simulink model "gap_generation_single_veh"  (R2019a)
settings: Solver=VariableStepAuto  StartTime=0.0  StopTime=35  FixedStep=0.1  MaxStep=0.05  RelTol=1e-3
libraries: simulink x21, powerlib_meascontrol x5, autolibshared x5
(part 1 of 3)
settings Model: Creator=fvall  LastModifiedBy=fvall

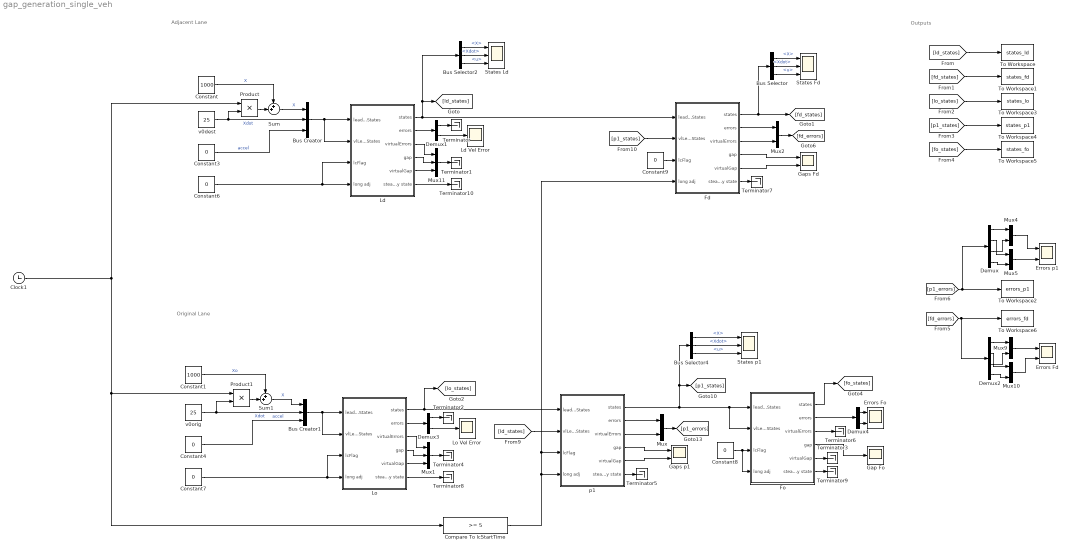
== system gap_generation_single_veh ==
  note: Original Lane
  note: Adjacent Lane
  note: Outputs
  Bus Creator : BusCreator  Inputs=3
  Bus Creator1 : BusCreator  Inputs=3
  Bus Selector : BusSelector  OutputSignals=X,Xdot,u
  Bus Selector2 : BusSelector  OutputSignals=X,Xdot,u
  Bus Selector4 : BusSelector  OutputSignals=X,Xdot,u
  Clock1 : Clock
  Compare To lcStartTime : simulink/Logic and Bit Operations/Compare To Constant  relop=>=  const=5  OutDataTypeStr=boolean
  Constant : Constant  Value=1000
  Constant1 : Constant  Value=1000
  Constant{3..4,6..9} (6 alike) : Constant  Value=0
  Demux : Demux
  Demux1 : Demux  Outputs=2
  Demux2 : Demux
  Demux3 : Demux  Outputs=2
  Demux4 : Demux  Outputs=2
  Errors Fd : Scope  NumInputPorts=2
  Errors Fo : Scope  NumInputPorts=2
  Errors p1 : Scope  NumInputPorts=2
  Fd : Subsystem  mask{m=2000, lf=2.5, lr=2.5, maxAcceleration=4, minAcceleration=-8, maxJerk=40, minJerk=-50, x0=20.2504, vx0=25, y0=3.6, h=0.63, d0=0.5004, minHeadwayError=-100, maxHeadwayError=3, velFilterGain=10, Kd=1.5652, Kp=2.2775, Ki=0.75, velKi=0.5, velKp=1.5, hFilterGain=0.5, vMin=16.25, l1=-10, maxComfAccel=2, minComfAccel=-2, maxComfJerk=10, minComfJerk=-10, hLc=1.9025, d0Lc=0.5004}
      mask prompts: m "autoblks_shared:autoblkVehBody3DofLat:blkPrm_m"; lf "autoblks_shared:autoblkVehBody3DofLat:blkPrm_a"; lr "autoblks_shared:autoblkVehBody3DofLat:blkPrm_b"; maxAcceleration "Max Acceleration"; minAcceleration "Min Acceleration"; maxJerk "Max Jerk"; minJerk "Min Jerk"; x0 "autoblks_shared:autoblkVehBody3DofLat:blkPrm_X_o"; vx0 "autoblks_shared:autoblkVehBody3DofLat:blkPrm_xdot_o"; y0 "autoblks_shared:autoblkVehBody3DofLat:blkPrm_Y_o"; h "Time Headway"; d0 "Standstill Gap"; minHeadwayError "Min Headway Error"; maxHeadwayError "Max Headway Error"; velFilterGain "Velocity Filter Gain"; hFilterGain "Headway filter Gain"; vMin "Min velocity"; l1 "ACC-v Headway Error Threshold"; maxComfAccel "Max Comf Accel"; minComfAccel "Min Comf Accel"; maxComfJerk "Max Comf Jerk"; minComfJerk "Min Comf Jerk"; hLc "Time Headway LC"; d0Lc "Standstill Gap LC"
      mask TypeOptions m: Vehicle Body 3DOF Single Track/m
      mask TypeOptions lf: Vehicle Body 3DOF Single Track/a
      mask TypeOptions lr: Vehicle Body 3DOF Single Track/b
      mask TypeOptions x0: Vehicle Body 3DOF Single Track/X_o
      mask TypeOptions vx0: Vehicle Body 3DOF Single Track/xdot_o
      mask TypeOptions y0: Vehicle Body 3DOF Single Track/Y_o
      mask TypeOptions h:
      | Regular Vehicle
      | Following/Headway error/h/Value
      mask TypeOptions d0:
      | Regular Vehicle
      | Following/Headway error/d0/Value
      mask TypeOptions hFilterGain:
      | Regular Vehicle
      | Following/Headway error/hFilterGain/Gain
      mask TypeOptions vMin:
      | Longitudinal Adjustments
      | for Lane Change/vMin/Value
      mask TypeOptions hLc:
      | Regular Vehicle
      | Following/Headway error/hLc/Value
      mask TypeOptions d0Lc:
      | Regular Vehicle
      | Following/Headway error/d0Lc/Value
      mask DialogControl DescGroupVar Prompt: 3DOF Vehicle with ACC
      mask DialogControl DescTextVar Prompt: Vehicle with ACC. The vehicle model is Simulink's 3DOF single track vehicle body. The controller is a PID with constant headway including headway error saturation and filtered leader velocity.
      mask DialogControl VehParams Prompt: Vehicle Parameters
      mask DialogControl m Prompt: Vehicle mass, m [kg]:
      mask DialogControl lf Prompt: Longitudinal distance from center of mass to front axle, a [m]:
      mask DialogControl lr Prompt: Longitudinal distance from center of mass to rear axle, b [m]:
      mask DialogControl InitStates Prompt: Initial State
      mask DialogControl x0 Prompt: Initial inertial frame longitudinal position, X_o [m]:
      mask DialogControl vx0 Prompt: Initial longitudinal velocity, xdot_o [m/s]:
      mask DialogControl y0 Prompt: Initial inertial frame lateral displacement, Y_o [m]:
      mask DialogControl Container3 Prompt: Veh Following Parameters
      mask DialogControl VirtualFollParams Prompt: Virtual Veh Following Parameters
      mask DialogControl LCParams Prompt: Lane Change Params
  Fo : Subsystem  mask{m=2000, lf=2.5, lr=2.5, maxAcceleration=4, minAcceleration=-8, maxJerk=40, minJerk=-50, x0=0, vx0=25, y0=0, h=0.63, d0=0.5004, minHeadwayError=-100, maxHeadwayError=3, velFilterGain=10, Kd=1.5652, Kp=2.2775, Ki=0.75, velKi=0.5, velKp=1.5, hFilterGain=0.5, vMin=16.25, l1=-10, maxComfAccel=2, minComfAccel=-2, maxComfJerk=10, minComfJerk=-10, hLc=1.9025, d0Lc=0.5004}
      mask prompts: m "autoblks_shared:autoblkVehBody3DofLat:blkPrm_m"; lf "autoblks_shared:autoblkVehBody3DofLat:blkPrm_a"; lr "autoblks_shared:autoblkVehBody3DofLat:blkPrm_b"; maxAcceleration "Max Acceleration"; minAcceleration "Min Acceleration"; maxJerk "Max Jerk"; minJerk "Min Jerk"; x0 "autoblks_shared:autoblkVehBody3DofLat:blkPrm_X_o"; vx0 "autoblks_shared:autoblkVehBody3DofLat:blkPrm_xdot_o"; y0 "autoblks_shared:autoblkVehBody3DofLat:blkPrm_Y_o"; h "Time Headway"; d0 "Standstill Gap"; minHeadwayError "Min Headway Error"; maxHeadwayError "Max Headway Error"; velFilterGain "Velocity Filter Gain"; hFilterGain "Headway filter Gain"; vMin "Min velocity"; l1 "ACC-v Headway Error Threshold"; maxComfAccel "Max Comf Accel"; minComfAccel "Min Comf Accel"; maxComfJerk "Max Comf Jerk"; minComfJerk "Min Comf Jerk"; hLc "Time Headway LC"; d0Lc "Standstill Gap LC"
      mask TypeOptions m: Vehicle Body 3DOF Single Track/m
      mask TypeOptions lf: Vehicle Body 3DOF Single Track/a
      mask TypeOptions lr: Vehicle Body 3DOF Single Track/b
      mask TypeOptions x0: Vehicle Body 3DOF Single Track/X_o
      mask TypeOptions vx0: Vehicle Body 3DOF Single Track/xdot_o
      mask TypeOptions y0: Vehicle Body 3DOF Single Track/Y_o
      mask TypeOptions h:
      | Regular Vehicle
      | Following/Headway error/h/Value
      mask TypeOptions d0:
      | Regular Vehicle
      | Following/Headway error/d0/Value
      mask TypeOptions hFilterGain:
      | Regular Vehicle
      | Following/Headway error/hFilterGain/Gain
      mask TypeOptions vMin:
      | Longitudinal Adjustments
      | for Lane Change/vMin/Value
      mask TypeOptions hLc:
      | Regular Vehicle
      | Following/Headway error/hLc/Value
      mask TypeOptions d0Lc:
      | Regular Vehicle
      | Following/Headway error/d0Lc/Value
      mask DialogControl DescGroupVar Prompt: 3DOF Vehicle with ACC
      mask DialogControl DescTextVar Prompt: Vehicle with ACC. The vehicle model is Simulink's 3DOF single track vehicle body. The controller is a PID with constant headway including headway error saturation and filtered leader velocity.
      mask DialogControl VehParams Prompt: Vehicle Parameters
      mask DialogControl m Prompt: Vehicle mass, m [kg]:
      mask DialogControl lf Prompt: Longitudinal distance from center of mass to front axle, a [m]:
      mask DialogControl lr Prompt: Longitudinal distance from center of mass to rear axle, b [m]:
      mask DialogControl InitStates Prompt: Initial State
      mask DialogControl x0 Prompt: Initial inertial frame longitudinal position, X_o [m]:
      mask DialogControl vx0 Prompt: Initial longitudinal velocity, xdot_o [m/s]:
      mask DialogControl y0 Prompt: Initial inertial frame lateral displacement, Y_o [m]:
      mask DialogControl Container3 Prompt: Veh Following Parameters
      mask DialogControl VirtualFollParams Prompt: Virtual Veh Following Parameters
      mask DialogControl LCParams Prompt: Lane Change Params
  Gap Fo : Scope
  Gaps Fd : Scope  NumInputPorts=2
  Gaps p1 : Scope  NumInputPorts=2
  Ld : Subsystem  mask{m=2000, lf=2.5, lr=2.5, maxAcceleration=4, minAcceleration=-8, maxJerk=40, minJerk=-50, x0=41.5008, vx0=25, y0=3.6, h=0.63, d0=0.5004, minHeadwayError=-100, maxHeadwayError=3, velFilterGain=10, Kd=1.5652, Kp=2.2775, Ki=0.75, velKi=0.5, velKp=1.5, hFilterGain=0.5, vMin=16.25, l1=-10, maxComfAccel=2, minComfAccel=-2, maxComfJerk=10, minComfJerk=-10, hLc=1.9025, d0Lc=0.5004}
      mask prompts: m "autoblks_shared:autoblkVehBody3DofLat:blkPrm_m"; lf "autoblks_shared:autoblkVehBody3DofLat:blkPrm_a"; lr "autoblks_shared:autoblkVehBody3DofLat:blkPrm_b"; maxAcceleration "Max Acceleration"; minAcceleration "Min Acceleration"; maxJerk "Max Jerk"; minJerk "Min Jerk"; x0 "autoblks_shared:autoblkVehBody3DofLat:blkPrm_X_o"; vx0 "autoblks_shared:autoblkVehBody3DofLat:blkPrm_xdot_o"; y0 "autoblks_shared:autoblkVehBody3DofLat:blkPrm_Y_o"; h "Time Headway"; d0 "Standstill Gap"; minHeadwayError "Min Headway Error"; maxHeadwayError "Max Headway Error"; velFilterGain "Velocity Filter Gain"; hFilterGain "Headway filter Gain"; vMin "Min velocity"; l1 "ACC-v Headway Error Threshold"; maxComfAccel "Max Comf Accel"; minComfAccel "Min Comf Accel"; maxComfJerk "Max Comf Jerk"; minComfJerk "Min Comf Jerk"; hLc "Time Headway LC"; d0Lc "Standstill Gap LC"
      mask TypeOptions m: Vehicle Body 3DOF Single Track/m
      mask TypeOptions lf: Vehicle Body 3DOF Single Track/a
      mask TypeOptions lr: Vehicle Body 3DOF Single Track/b
      mask TypeOptions x0: Vehicle Body 3DOF Single Track/X_o
      mask TypeOptions vx0: Vehicle Body 3DOF Single Track/xdot_o
      mask TypeOptions y0: Vehicle Body 3DOF Single Track/Y_o
      mask TypeOptions h:
      | Regular Vehicle
      | Following/Headway error/h/Value
      mask TypeOptions d0:
      | Regular Vehicle
      | Following/Headway error/d0/Value
      mask TypeOptions hFilterGain:
      | Regular Vehicle
      | Following/Headway error/hFilterGain/Gain
      mask TypeOptions vMin:
      | Longitudinal Adjustments
      | for Lane Change/vMin/Value
      mask TypeOptions hLc:
      | Regular Vehicle
      | Following/Headway error/hLc/Value
      mask TypeOptions d0Lc:
      | Regular Vehicle
      | Following/Headway error/d0Lc/Value
      mask DialogControl DescGroupVar Prompt: 3DOF Vehicle with ACC
      mask DialogControl DescTextVar Prompt: Vehicle with ACC. The vehicle model is Simulink's 3DOF single track vehicle body. The controller is a PID with constant headway including headway error saturation and filtered leader velocity.
      mask DialogControl VehParams Prompt: Vehicle Parameters
      mask DialogControl m Prompt: Vehicle mass, m [kg]:
      mask DialogControl lf Prompt: Longitudinal distance from center of mass to front axle, a [m]:
      mask DialogControl lr Prompt: Longitudinal distance from center of mass to rear axle, b [m]:
      mask DialogControl InitStates Prompt: Initial State
      mask DialogControl x0 Prompt: Initial inertial frame longitudinal position, X_o [m]:
      mask DialogControl vx0 Prompt: Initial longitudinal velocity, xdot_o [m/s]:
      mask DialogControl y0 Prompt: Initial inertial frame lateral displacement, Y_o [m]:
      mask DialogControl Container3 Prompt: Veh Following Parameters
      mask DialogControl VirtualFollParams Prompt: Virtual Veh Following Parameters
      mask DialogControl LCParams Prompt: Lane Change Params
  Ld Vel Error : Scope
  Lo : Subsystem  mask{m=2000, lf=2.5, lr=2.5, maxAcceleration=4, minAcceleration=-8, maxJerk=40, minJerk=-50, x0=42.5008, vx0=25, y0=0, h=0.63, d0=0.5004, minHeadwayError=-100, maxHeadwayError=3, velFilterGain=10, Kd=1.5652, Kp=2.2775, Ki=0.75, velKi=0.5, velKp=1.5, hFilterGain=0.5, vMin=16.25, l1=-10, maxComfAccel=2, minComfAccel=-2, maxComfJerk=10, minComfJerk=-10, hLc=1.9025, d0Lc=0.5004}
      mask prompts: m "autoblks_shared:autoblkVehBody3DofLat:blkPrm_m"; lf "autoblks_shared:autoblkVehBody3DofLat:blkPrm_a"; lr "autoblks_shared:autoblkVehBody3DofLat:blkPrm_b"; maxAcceleration "Max Acceleration"; minAcceleration "Min Acceleration"; maxJerk "Max Jerk"; minJerk "Min Jerk"; x0 "autoblks_shared:autoblkVehBody3DofLat:blkPrm_X_o"; vx0 "autoblks_shared:autoblkVehBody3DofLat:blkPrm_xdot_o"; y0 "autoblks_shared:autoblkVehBody3DofLat:blkPrm_Y_o"; h "Time Headway"; d0 "Standstill Gap"; minHeadwayError "Min Headway Error"; maxHeadwayError "Max Headway Error"; velFilterGain "Velocity Filter Gain"; hFilterGain "Headway filter Gain"; vMin "Min velocity"; l1 "ACC-v Headway Error Threshold"; maxComfAccel "Max Comf Accel"; minComfAccel "Min Comf Accel"; maxComfJerk "Max Comf Jerk"; minComfJerk "Min Comf Jerk"; hLc "Time Headway LC"; d0Lc "Standstill Gap LC"
      mask TypeOptions m: Vehicle Body 3DOF Single Track/m
      mask TypeOptions lf: Vehicle Body 3DOF Single Track/a
      mask TypeOptions lr: Vehicle Body 3DOF Single Track/b
      mask TypeOptions x0: Vehicle Body 3DOF Single Track/X_o
      mask TypeOptions vx0: Vehicle Body 3DOF Single Track/xdot_o
      mask TypeOptions y0: Vehicle Body 3DOF Single Track/Y_o
      mask TypeOptions h:
      | Regular Vehicle
      | Following/Headway error/h/Value
      mask TypeOptions d0:
      | Regular Vehicle
      | Following/Headway error/d0/Value
      mask TypeOptions hFilterGain:
      | Regular Vehicle
      | Following/Headway error/hFilterGain/Gain
      mask TypeOptions vMin:
      | Longitudinal Adjustments
      | for Lane Change/vMin/Value
      mask TypeOptions hLc:
      | Regular Vehicle
      | Following/Headway error/hLc/Value
      mask TypeOptions d0Lc:
      | Regular Vehicle
      | Following/Headway error/d0Lc/Value
      mask DialogControl DescGroupVar Prompt: 3DOF Vehicle with ACC
      mask DialogControl DescTextVar Prompt: Vehicle with ACC. The vehicle model is Simulink's 3DOF single track vehicle body. The controller is a PID with constant headway including headway error saturation and filtered leader velocity.
      mask DialogControl VehParams Prompt: Vehicle Parameters
      mask DialogControl m Prompt: Vehicle mass, m [kg]:
      mask DialogControl lf Prompt: Longitudinal distance from center of mass to front axle, a [m]:
      mask DialogControl lr Prompt: Longitudinal distance from center of mass to rear axle, b [m]:
      mask DialogControl InitStates Prompt: Initial State
      mask DialogControl x0 Prompt: Initial inertial frame longitudinal position, X_o [m]:
      mask DialogControl vx0 Prompt: Initial longitudinal velocity, xdot_o [m/s]:
      mask DialogControl y0 Prompt: Initial inertial frame lateral displacement, Y_o [m]:
      mask DialogControl Container3 Prompt: Veh Following Parameters
      mask DialogControl VirtualFollParams Prompt: Virtual Veh Following Parameters
      mask DialogControl LCParams Prompt: Lane Change Params
  Lo Vel Error : Scope
  Mux{,2,4..5,9..10} (6 alike) : Mux  Inputs=2
  Mux1 : Mux  Inputs=3
  Mux11 : Mux  Inputs=3
  Product : Product
  Product1 : Product
  States Fd : Scope  NumInputPorts=3
  States Ld : Scope  NumInputPorts=3
  States p1 : Scope  NumInputPorts=3
  Sum : Sum  Inputs=++|
  Sum1 : Sum  Inputs=++|
  Terminator{,1..10} (11 alike) : Terminator
  To Workspace : ToWorkspace  VariableName=states_ld  SampleTime=-1
  To Workspace1 : ToWorkspace  VariableName=states_fd  SampleTime=-1
  To Workspace2 : ToWorkspace  VariableName=errors_p1  SampleTime=-1
  To Workspace3 : ToWorkspace  VariableName=states_lo  SampleTime=-1
  To Workspace4 : ToWorkspace  VariableName=states_p1  SampleTime=-1
  To Workspace5 : ToWorkspace  VariableName=states_fo  SampleTime=-1
  To Workspace6 : ToWorkspace  VariableName=errors_fd  SampleTime=-1
  p1 : Subsystem  mask{m=2000, lf=2.5, lr=2.5, maxAcceleration=4, minAcceleration=-8, maxJerk=40, minJerk=-50, x0=21.2504, vx0=25, y0=0, h=0.63, d0=0.5004, minHeadwayError=-100, maxHeadwayError=3, velFilterGain=10, Kd=1.5652, Kp=2.2775, Ki=0.75, velKi=0.5, velKp=1.5, hFilterGain=0.5, vMin=16.25, l1=-10, maxComfAccel=2, minComfAccel=-2, maxComfJerk=10, minComfJerk=-10, hLc=1.9025, d0Lc=0.5004}
      mask prompts: m "autoblks_shared:autoblkVehBody3DofLat:blkPrm_m"; lf "autoblks_shared:autoblkVehBody3DofLat:blkPrm_a"; lr "autoblks_shared:autoblkVehBody3DofLat:blkPrm_b"; maxAcceleration "Max Acceleration"; minAcceleration "Min Acceleration"; maxJerk "Max Jerk"; minJerk "Min Jerk"; x0 "autoblks_shared:autoblkVehBody3DofLat:blkPrm_X_o"; vx0 "autoblks_shared:autoblkVehBody3DofLat:blkPrm_xdot_o"; y0 "autoblks_shared:autoblkVehBody3DofLat:blkPrm_Y_o"; h "Time Headway"; d0 "Standstill Gap"; minHeadwayError "Min Headway Error"; maxHeadwayError "Max Headway Error"; velFilterGain "Velocity Filter Gain"; hFilterGain "Headway filter Gain"; vMin "Min velocity"; l1 "ACC-v Headway Error Threshold"; maxComfAccel "Max Comf Accel"; minComfAccel "Min Comf Accel"; maxComfJerk "Max Comf Jerk"; minComfJerk "Min Comf Jerk"; hLc "Time Headway LC"; d0Lc "Standstill Gap LC"
      mask TypeOptions m: Vehicle Body 3DOF Single Track/m
      mask TypeOptions lf: Vehicle Body 3DOF Single Track/a
      mask TypeOptions lr: Vehicle Body 3DOF Single Track/b
      mask TypeOptions x0: Vehicle Body 3DOF Single Track/X_o
      mask TypeOptions vx0: Vehicle Body 3DOF Single Track/xdot_o
      mask TypeOptions y0: Vehicle Body 3DOF Single Track/Y_o
      mask TypeOptions h:
      | Regular Vehicle
      | Following/Headway error/h/Value
      mask TypeOptions d0:
      | Regular Vehicle
      | Following/Headway error/d0/Value
      mask TypeOptions hFilterGain:
      | Regular Vehicle
      | Following/Headway error/hFilterGain/Gain
      mask TypeOptions vMin:
      | Longitudinal Adjustments
      | for Lane Change/vMin/Value
      mask TypeOptions hLc:
      | Regular Vehicle
      | Following/Headway error/hLc/Value
      mask TypeOptions d0Lc:
      | Regular Vehicle
      | Following/Headway error/d0Lc/Value
      mask DialogControl DescGroupVar Prompt: 3DOF Vehicle with ACC
      mask DialogControl DescTextVar Prompt: Vehicle with ACC. The vehicle model is Simulink's 3DOF single track vehicle body. The controller is a PID with constant headway including headway error saturation and filtered leader velocity.
      mask DialogControl VehParams Prompt: Vehicle Parameters
      mask DialogControl m Prompt: Vehicle mass, m [kg]:
      mask DialogControl lf Prompt: Longitudinal distance from center of mass to front axle, a [m]:
      mask DialogControl lr Prompt: Longitudinal distance from center of mass to rear axle, b [m]:
      mask DialogControl InitStates Prompt: Initial State
      mask DialogControl x0 Prompt: Initial inertial frame longitudinal position, X_o [m]:
      mask DialogControl vx0 Prompt: Initial longitudinal velocity, xdot_o [m/s]:
      mask DialogControl y0 Prompt: Initial inertial frame lateral displacement, Y_o [m]:
      mask DialogControl Container3 Prompt: Veh Following Parameters
      mask DialogControl VirtualFollParams Prompt: Virtual Veh Following Parameters
      mask DialogControl LCParams Prompt: Lane Change Params
  v0dest : Constant  Value=25
  v0orig : Constant  Value=25
  wires:
  Clock1/1 -> Product/1, Compare To lcStartTime/1, Product1/1
  Lo/1(states) -> p1/1(leaderStates), [lo_states]
  Bus Selector4/3 -> States p1/3  "<u>"
  Bus Selector4/2 -> States p1/2  "<Xdot>"
  Bus Selector4/1 -> States p1/1  "<X>"
  p1/2(errors) -> Mux/1
  Ld/2(errors) -> Demux1/1
  Bus Selector2/3 -> States Ld/3  "<u>"
  Fd/6(steady state) -> Terminator7/1
  Fd/3(virtualErrors) -> Mux2/2
  Fd/5(virtualGap) -> Gaps Fd/2
  Fd/1(states) -> [fd_states], Bus Selector/1
  Ld/3(virtualErrors) -> Mux11/1
  Fd/4(gap) -> Gaps Fd/1
  Mux11/1 -> Terminator1/1
  Fd/2(errors) -> Mux2/1
  Demux1/2 -> Ld Vel Error/1
  Bus Selector2/2 -> States Ld/2  "<Xdot>"
  Bus Selector2/1 -> States Ld/1  "<X>"
  Ld/6(steady state) -> Terminator10/1
  Bus Selector/1 -> States Fd/1  "<X>"
  [p1_states] -> Fd/2(vlLeaderStates)
  Constant9/1 -> Fd/3(lcFlag)
  Ld/5(virtualGap) -> Mux11/3
  Bus Selector/3 -> States Fd/3  "<u>"
  Constant6/1 -> Ld/4(long adj), Ld/3(lcFlag)
  Ld/4(gap) -> Mux11/2
  Bus Selector/2 -> States Fd/2  "<Xdot>"
  Ld/1(states) -> Fd/1(leaderStates), Bus Selector2/1, [ld_states]
  v0dest/1 -> Product/2, Bus Creator/2  "Xdot"
  Constant3/1 -> Bus Creator/3  "accel"
  Mux2/1 -> [fd_errors]
  Sum/1 -> Bus Creator/1  "X"
  Demux1/1 -> Terminator/1
  Bus Creator/1 -> Ld/1(leaderStates), Ld/2(vlLeaderStates)
  Bus Creator1/1 -> Lo/2(vlLeaderStates), Lo/1(leaderStates)
  Constant7/1 -> Lo/3(lcFlag), Lo/4(long adj)
  v0orig/1 -> Bus Creator1/2, Product1/2  "Xdot"
  Constant4/1 -> Bus Creator1/3  "accel"
  Sum1/1 -> Bus Creator1/1  "X"
  Fo/5(virtualGap) -> Terminator3/1
  Fo/2(errors) -> Demux4/1
  Fo/4(gap) -> Gap Fo/1
  Demux4/2 -> Errors Fo/2
  Constant8/1 -> Fo/4(long adj), Fo/3(lcFlag)
  Demux4/1 -> Errors Fo/1
  Fo/1(states) -> [fo_states]
  p1/1(states) -> Bus Selector4/1, [p1_states], Fo/2(vlLeaderStates), Fo/1(leaderStates)
  [ld_states] -> p1/2(vlLeaderStates)
  Compare To lcStartTime/1 -> p1/4(long adj), p1/3(lcFlag), Fd/4(long adj)
  p1/4(gap) -> Gaps p1/1
  [fd_states] -> To Workspace1/1
  [lo_states] -> To Workspace3/1
  Mux10/1 -> Errors Fd/2
  Mux4/1 -> Errors p1/1
  Demux/2 -> Mux5/1
  Mux9/1 -> Errors Fd/1
  Demux/3 -> Mux4/2
  Demux/1 -> Mux4/1
  Mux5/1 -> Errors p1/2
  Demux2/2 -> Mux10/1
  Demux2/3 -> Mux9/2
  [p1_errors] -> To Workspace2/1, Demux/1
  [fd_errors] -> Demux2/1, To Workspace6/1
  [p1_states] -> To Workspace4/1
  Demux2/4 -> Mux10/2
  [ld_states] -> To Workspace/1
  Demux/4 -> Mux5/2
  [fo_states] -> To Workspace5/1
  Demux2/1 -> Mux9/1
  Mux/1 -> [p1_errors]
  p1/3(virtualErrors) -> Mux/2
  p1/6(steady state) -> Terminator5/1
  Fo/6(steady state) -> Terminator9/1
  Product/1 -> Sum/2
  Constant/1 -> Sum/1  "X"
  Product1/1 -> Sum1/2
  Constant1/1 -> Sum1/1  "Xo"
  p1/5(virtualGap) -> Gaps p1/2
  Mux1/1 -> Terminator4/1
  Lo/4(gap) -> Mux1/2
  Lo/3(virtualErrors) -> Mux1/1
  Lo/2(errors) -> Demux3/1
  Demux3/2 -> Lo Vel Error/1
  Lo/5(virtualGap) -> Mux1/3
  Lo/6(steady state) -> Terminator8/1
  Demux3/1 -> Terminator2/1
  Fo/3(virtualErrors) -> Terminator6/1

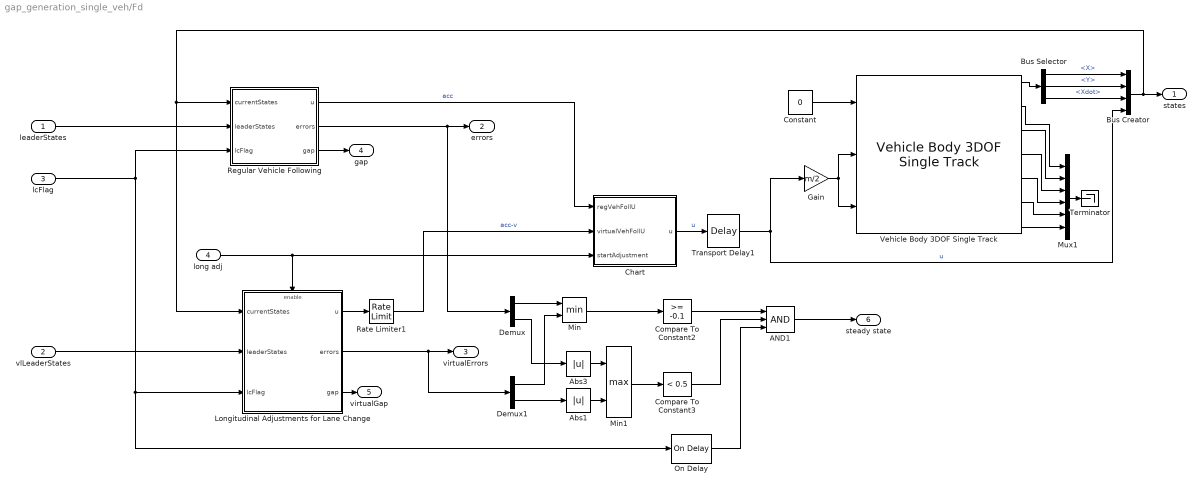
== system gap_generation_single_veh/Fd ==
  leaderStates : Inport
  vlLeaderStates : Inport  Port=2
  lcFlag : Inport  Port=3
  long adj : Inport  Port=4
  AND1 : Logic  Inputs=3  IconShape=distinctive  AllPortsSameDT=off  OutDataTypeStr=boolean
  Abs1 : Abs
  Abs3 : Abs
  Bus Creator : BusCreator  Inputs=4
  Bus Selector : BusSelector  OutputSignals=InertFrm.RearAxl.Disp.X,InertFrm.RearAxl.Disp.Y,InertFrm.RearAxl.Vel.Xdot
  Chart : Stateflow chart  BlockKeywords=__PRM__SERIALIZED__DATA__:Stateflow Chart,Stateflow Diagram  TreatAsAtomicUnit=on
  Compare To Constant2 : simulink/Logic and Bit Operations/Compare To Constant  relop=>=  const=-0.1  OutDataTypeStr=boolean
  Compare To Constant3 : simulink/Logic and Bit Operations/Compare To Constant  relop=<  const=0.5  OutDataTypeStr=boolean
  Constant : Constant  Value=0
  Demux : Demux  Outputs=2
  Demux1 : Demux  Outputs=2
  Gain : Gain  Gain=m/2
  Longitudinal Adjustments for Lane Change : Subsystem  TreatAsAtomicUnit=on
  Min : MinMax  Inputs=2
  Min1 : MinMax  Function=max  Inputs=2
  Mux1 : Mux  Inputs=6
  On Delay : powerlib_meascontrol/Logic/On Delay  DelayType=On delay  delay=1  ic=0  Ts=0
      settings: SourceProductName=Simscape Electrical
  Rate Limiter1 : RateLimiter  RisingSlewLimit=10  FallingSlewLimit=-10  SampleTimeMode=inherited
  Regular Vehicle Following : Subsystem
  Terminator : Terminator
  Transport Delay1 : TransportDelay  DelayTime=0.01
  Vehicle Body 3DOF Single Track : autolibshared/Vehicle Body 3DOF Single Track  trackMode=Single (bicycle)  inputMode=External longitudinal forces  frontSteerMode=on  rearSteerMode=off  windMode=off  muMode=off  extFMode=off  extMMode=off  extXo=off  extpsio=off  extxdoto=off  extro=off  extYo=off  extTamb=off  extydoto=off  aMode=2  NF=2  NR=2  m=m  a=lf  b=lr  h=0.35  X_o=x0  xdot_o=vx0  CalphaMode=off  sigmaMode=on  d=0  w=[1.4,1.4]  Cy_f=12e3  Cy_r=11e3  sigma_f=.1  sigma_r=.1  alpha_f_brk=[-.1 .1]  Cy_f_data=[-9e3 9e3]  alpha_r_brk=[-.1 .1]  Cy_r_data=[-9e3 9e3]  Y_o=y0  ydot_o=0  Izz=4000  psi_o=0  r_o=0  Af=2  Cd=.3  Cl=.1  Cpm=.1  beta_w=[0:0.01:0.3]  Cs=[0:0.03:0.9]  Cym=[0:0.01:0.3]  Pabs=101325  Tair=273  g=9.81  mu=1  xdot_tol=.01  Fznom=5000  Fxtire_sat=7e4  Fytire_sat=7e4  longOff=0  latOff=0  vertOff=0  wrapAng=off
      settings: SourceProductName=Powertrain Blockset  SourceProductBaseCode=PW
  states : Outport
  errors : Outport  Port=2
  virtualErrors : Outport  Port=3
  gap : Outport  Port=4
  virtualGap : Outport  Port=5
  steady state : Outport  Port=6
  wires:
  Bus Selector/3 -> Bus Creator/3  "<Xdot>"
  Bus Selector/1 -> Bus Creator/1  "<X>"
  Gain/1 -> Vehicle Body 3DOF Single Track/3, Vehicle Body 3DOF Single Track/2
  Vehicle Body 3DOF Single Track/1 -> Bus Selector/1
  Vehicle Body 3DOF Single Track/4 -> Mux1/3
  Vehicle Body 3DOF Single Track/3 -> Mux1/2
  Vehicle Body 3DOF Single Track/2 -> Mux1/1
  Vehicle Body 3DOF Single Track/5 -> Mux1/4
  Vehicle Body 3DOF Single Track/6 -> Mux1/5
  Vehicle Body 3DOF Single Track/7 -> Mux1/6
  Mux1/1 -> Terminator/1
  Regular Vehicle Following/3(gap) -> gap/1
  Bus Creator/1 -> states/1, Regular Vehicle Following/1(currentStates), Longitudinal Adjustments for Lane Change/1(currentStates)
  leaderStates/1 -> Regular Vehicle Following/2(leaderStates)
  vlLeaderStates/1 -> Longitudinal Adjustments for Lane Change/2(leaderStates)
  lcFlag/1 -> Regular Vehicle Following/3(lcFlag), Longitudinal Adjustments for Lane Change/3(lcFlag), On Delay/1
  Longitudinal Adjustments for Lane Change/3(gap) -> virtualGap/1
  long adj/1 -> Chart/3(startAdjustment), Longitudinal Adjustments for Lane Change/Enable
  On Delay/1 -> AND1/3
  AND1/1 -> steady state/1
  Longitudinal Adjustments for Lane Change/1(u) -> Rate Limiter1/1
  Regular Vehicle Following/1(u) -> Chart/1(regVehFollU)  "acc"
  Rate Limiter1/1 -> Chart/2(virtualVehFollU)  "acc-v"
  Chart/1(u) -> Transport Delay1/1  "u"
  Transport Delay1/1 -> Bus Creator/4, Gain/1  "u"
  Regular Vehicle Following/2(errors) -> errors/1, Demux/1
  Min/1 -> Compare To Constant2/1
  Demux/1 -> Min/1
  Demux1/1 -> Min/2
  Demux/2 -> Abs3/1
  Demux1/2 -> Abs1/1
  Compare To Constant2/1 -> AND1/1
  Compare To Constant3/1 -> AND1/2
  Min1/1 -> Compare To Constant3/1
  Longitudinal Adjustments for Lane Change/2(errors) -> virtualErrors/1, Demux1/1
  Abs3/1 -> Min1/1
  Abs1/1 -> Min1/2
  Bus Selector/2 -> Bus Creator/2  "<Y>"
  Constant/1 -> Vehicle Body 3DOF Single Track/1

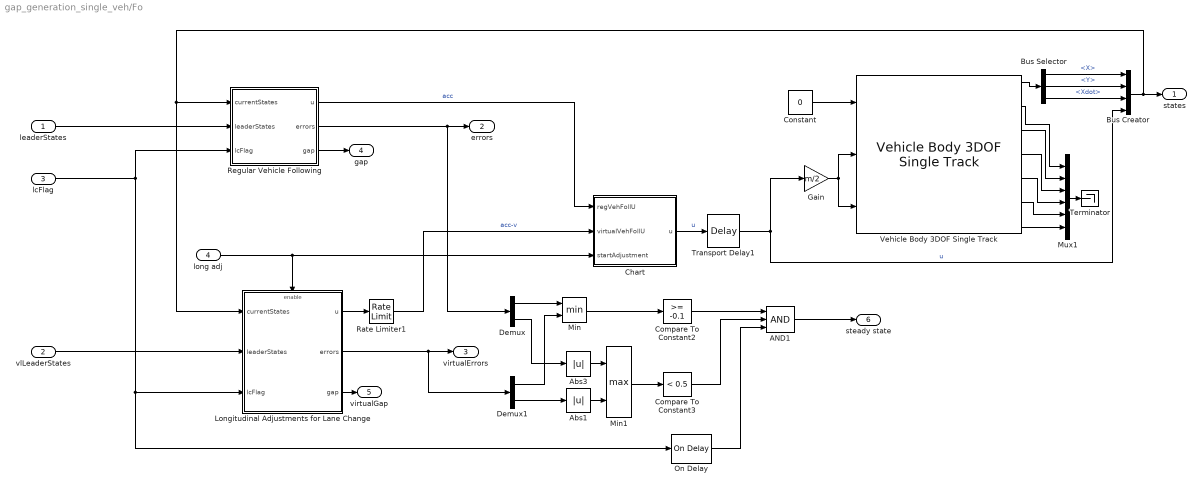
== system gap_generation_single_veh/Fo ==
  leaderStates : Inport
  vlLeaderStates : Inport  Port=2
  lcFlag : Inport  Port=3
  long adj : Inport  Port=4
  AND1 : Logic  Inputs=3  IconShape=distinctive  AllPortsSameDT=off  OutDataTypeStr=boolean
  Abs1 : Abs
  Abs3 : Abs
  Bus Creator : BusCreator  Inputs=4
  Bus Selector : BusSelector  OutputSignals=InertFrm.RearAxl.Disp.X,InertFrm.RearAxl.Disp.Y,InertFrm.RearAxl.Vel.Xdot
  Chart : Stateflow chart  BlockKeywords=__PRM__SERIALIZED__DATA__:Stateflow Chart,Stateflow Diagram  TreatAsAtomicUnit=on
  Compare To Constant2 : simulink/Logic and Bit Operations/Compare To Constant  relop=>=  const=-0.1  OutDataTypeStr=boolean
  Compare To Constant3 : simulink/Logic and Bit Operations/Compare To Constant  relop=<  const=0.5  OutDataTypeStr=boolean
  Constant : Constant  Value=0
  Demux : Demux  Outputs=2
  Demux1 : Demux  Outputs=2
  Gain : Gain  Gain=m/2
  Longitudinal Adjustments for Lane Change : Subsystem  TreatAsAtomicUnit=on
  Min : MinMax  Inputs=2
  Min1 : MinMax  Function=max  Inputs=2
  Mux1 : Mux  Inputs=6
  On Delay : powerlib_meascontrol/Logic/On Delay  DelayType=On delay  delay=1  ic=0  Ts=0
      settings: SourceProductName=Simscape Electrical
  Rate Limiter1 : RateLimiter  RisingSlewLimit=10  FallingSlewLimit=-10  SampleTimeMode=inherited
  Regular Vehicle Following : Subsystem
  Terminator : Terminator
  Transport Delay1 : TransportDelay  DelayTime=0.01
  Vehicle Body 3DOF Single Track : autolibshared/Vehicle Body 3DOF Single Track  trackMode=Single (bicycle)  inputMode=External longitudinal forces  frontSteerMode=on  rearSteerMode=off  windMode=off  muMode=off  extFMode=off  extMMode=off  extXo=off  extpsio=off  extxdoto=off  extro=off  extYo=off  extTamb=off  extydoto=off  aMode=2  NF=2  NR=2  m=m  a=lf  b=lr  h=0.35  X_o=x0  xdot_o=vx0  CalphaMode=off  sigmaMode=on  d=0  w=[1.4,1.4]  Cy_f=12e3  Cy_r=11e3  sigma_f=.1  sigma_r=.1  alpha_f_brk=[-.1 .1]  Cy_f_data=[-9e3 9e3]  alpha_r_brk=[-.1 .1]  Cy_r_data=[-9e3 9e3]  Y_o=y0  ydot_o=0  Izz=4000  psi_o=0  r_o=0  Af=2  Cd=.3  Cl=.1  Cpm=.1  beta_w=[0:0.01:0.3]  Cs=[0:0.03:0.9]  Cym=[0:0.01:0.3]  Pabs=101325  Tair=273  g=9.81  mu=1  xdot_tol=.01  Fznom=5000  Fxtire_sat=7e4  Fytire_sat=7e4  longOff=0  latOff=0  vertOff=0  wrapAng=off
      settings: SourceProductName=Powertrain Blockset  SourceProductBaseCode=PW
  states : Outport
  errors : Outport  Port=2
  virtualErrors : Outport  Port=3
  gap : Outport  Port=4
  virtualGap : Outport  Port=5
  steady state : Outport  Port=6
  wires:
  Constant/1 -> Vehicle Body 3DOF Single Track/1
  Bus Selector/2 -> Bus Creator/2  "<Y>"
  Abs1/1 -> Min1/2
  Abs3/1 -> Min1/1
  Longitudinal Adjustments for Lane Change/2(errors) -> Demux1/1, virtualErrors/1
  Min1/1 -> Compare To Constant3/1
  Compare To Constant3/1 -> AND1/2
  Compare To Constant2/1 -> AND1/1
  Demux1/2 -> Abs1/1
  Demux/2 -> Abs3/1
  Demux1/1 -> Min/2
  Demux/1 -> Min/1
  Min/1 -> Compare To Constant2/1
  Regular Vehicle Following/2(errors) -> Demux/1, errors/1
  Transport Delay1/1 -> Gain/1, Bus Creator/4  "u"
  Chart/1(u) -> Transport Delay1/1  "u"
  Rate Limiter1/1 -> Chart/2(virtualVehFollU)  "acc-v"
  Regular Vehicle Following/1(u) -> Chart/1(regVehFollU)  "acc"
  Longitudinal Adjustments for Lane Change/1(u) -> Rate Limiter1/1
  AND1/1 -> steady state/1
  On Delay/1 -> AND1/3
  long adj/1 -> Longitudinal Adjustments for Lane Change/Enable, Chart/3(startAdjustment)
  Longitudinal Adjustments for Lane Change/3(gap) -> virtualGap/1
  lcFlag/1 -> On Delay/1, Longitudinal Adjustments for Lane Change/3(lcFlag), Regular Vehicle Following/3(lcFlag)
  vlLeaderStates/1 -> Longitudinal Adjustments for Lane Change/2(leaderStates)
  leaderStates/1 -> Regular Vehicle Following/2(leaderStates)
  Bus Creator/1 -> Longitudinal Adjustments for Lane Change/1(currentStates), Regular Vehicle Following/1(currentStates), states/1
  Regular Vehicle Following/3(gap) -> gap/1
  Mux1/1 -> Terminator/1
  Vehicle Body 3DOF Single Track/7 -> Mux1/6
  Vehicle Body 3DOF Single Track/6 -> Mux1/5
  Vehicle Body 3DOF Single Track/5 -> Mux1/4
  Vehicle Body 3DOF Single Track/2 -> Mux1/1
  Vehicle Body 3DOF Single Track/3 -> Mux1/2
  Vehicle Body 3DOF Single Track/4 -> Mux1/3
  Vehicle Body 3DOF Single Track/1 -> Bus Selector/1
  Gain/1 -> Vehicle Body 3DOF Single Track/2, Vehicle Body 3DOF Single Track/3
  Bus Selector/1 -> Bus Creator/1  "<X>"
  Bus Selector/3 -> Bus Creator/3  "<Xdot>"

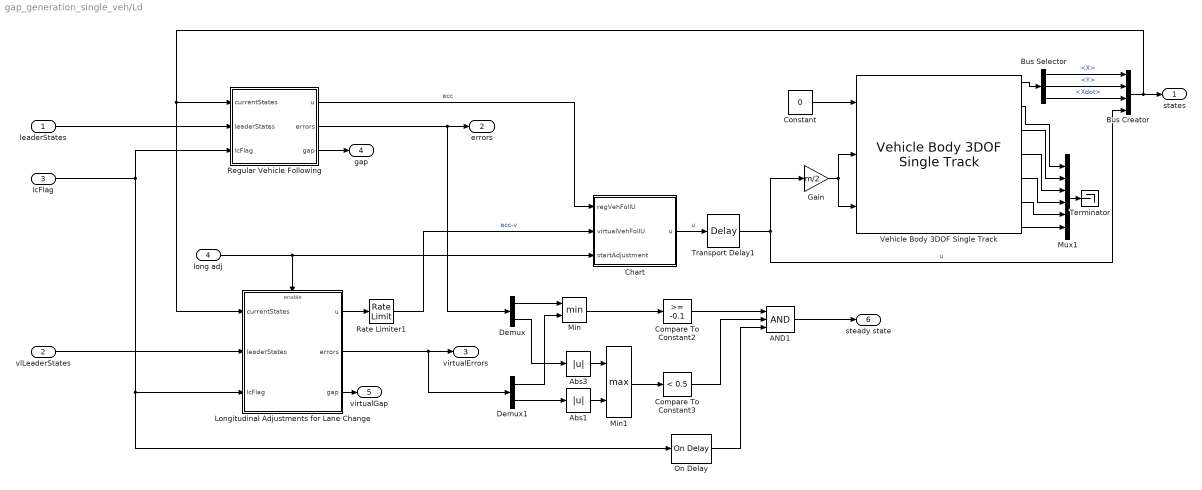
== system gap_generation_single_veh/Ld ==
  leaderStates : Inport
  vlLeaderStates : Inport  Port=2
  lcFlag : Inport  Port=3
  long adj : Inport  Port=4
  AND1 : Logic  Inputs=3  IconShape=distinctive  AllPortsSameDT=off  OutDataTypeStr=boolean
  Abs1 : Abs
  Abs3 : Abs
  Bus Creator : BusCreator  Inputs=4
  Bus Selector : BusSelector  OutputSignals=InertFrm.RearAxl.Disp.X,InertFrm.RearAxl.Disp.Y,InertFrm.RearAxl.Vel.Xdot
  Chart : Stateflow chart  BlockKeywords=__PRM__SERIALIZED__DATA__:Stateflow Chart,Stateflow Diagram  TreatAsAtomicUnit=on
  Compare To Constant2 : simulink/Logic and Bit Operations/Compare To Constant  relop=>=  const=-0.1  OutDataTypeStr=boolean
  Compare To Constant3 : simulink/Logic and Bit Operations/Compare To Constant  relop=<  const=0.5  OutDataTypeStr=boolean
  Constant : Constant  Value=0
  Demux : Demux  Outputs=2
  Demux1 : Demux  Outputs=2
  Gain : Gain  Gain=m/2
  Longitudinal Adjustments for Lane Change : Subsystem  TreatAsAtomicUnit=on
  Min : MinMax  Inputs=2
  Min1 : MinMax  Function=max  Inputs=2
  Mux1 : Mux  Inputs=6
  On Delay : powerlib_meascontrol/Logic/On Delay  DelayType=On delay  delay=1  ic=0  Ts=0
      settings: SourceProductName=Simscape Electrical
  Rate Limiter1 : RateLimiter  RisingSlewLimit=10  FallingSlewLimit=-10  SampleTimeMode=inherited
  Regular Vehicle Following : Subsystem
  Terminator : Terminator
  Transport Delay1 : TransportDelay  DelayTime=0.01
  Vehicle Body 3DOF Single Track : autolibshared/Vehicle Body 3DOF Single Track  trackMode=Single (bicycle)  inputMode=External longitudinal forces  frontSteerMode=on  rearSteerMode=off  windMode=off  muMode=off  extFMode=off  extMMode=off  extXo=off  extpsio=off  extxdoto=off  extro=off  extYo=off  extTamb=off  extydoto=off  aMode=2  NF=2  NR=2  m=m  a=lf  b=lr  h=0.35  X_o=x0  xdot_o=vx0  CalphaMode=off  sigmaMode=on  d=0  w=[1.4,1.4]  Cy_f=12e3  Cy_r=11e3  sigma_f=.1  sigma_r=.1  alpha_f_brk=[-.1 .1]  Cy_f_data=[-9e3 9e3]  alpha_r_brk=[-.1 .1]  Cy_r_data=[-9e3 9e3]  Y_o=y0  ydot_o=0  Izz=4000  psi_o=0  r_o=0  Af=2  Cd=.3  Cl=.1  Cpm=.1  beta_w=[0:0.01:0.3]  Cs=[0:0.03:0.9]  Cym=[0:0.01:0.3]  Pabs=101325  Tair=273  g=9.81  mu=1  xdot_tol=.01  Fznom=5000  Fxtire_sat=7e4  Fytire_sat=7e4  longOff=0  latOff=0  vertOff=0  wrapAng=off
      settings: SourceProductName=Powertrain Blockset  SourceProductBaseCode=PW
  states : Outport
  errors : Outport  Port=2
  virtualErrors : Outport  Port=3
  gap : Outport  Port=4
  virtualGap : Outport  Port=5
  steady state : Outport  Port=6
  wires:
  Constant/1 -> Vehicle Body 3DOF Single Track/1
  Bus Selector/2 -> Bus Creator/2  "<Y>"
  Abs1/1 -> Min1/2
  Abs3/1 -> Min1/1
  Longitudinal Adjustments for Lane Change/2(errors) -> Demux1/1, virtualErrors/1
  Min1/1 -> Compare To Constant3/1
  Compare To Constant3/1 -> AND1/2
  Compare To Constant2/1 -> AND1/1
  Demux1/2 -> Abs1/1
  Demux/2 -> Abs3/1
  Demux1/1 -> Min/2
  Demux/1 -> Min/1
  Min/1 -> Compare To Constant2/1
  Regular Vehicle Following/2(errors) -> Demux/1, errors/1
  Transport Delay1/1 -> Gain/1, Bus Creator/4  "u"
  Chart/1(u) -> Transport Delay1/1  "u"
  Rate Limiter1/1 -> Chart/2(virtualVehFollU)  "acc-v"
  Regular Vehicle Following/1(u) -> Chart/1(regVehFollU)  "acc"
  Longitudinal Adjustments for Lane Change/1(u) -> Rate Limiter1/1
  AND1/1 -> steady state/1
  On Delay/1 -> AND1/3
  long adj/1 -> Longitudinal Adjustments for Lane Change/Enable, Chart/3(startAdjustment)
  Longitudinal Adjustments for Lane Change/3(gap) -> virtualGap/1
  lcFlag/1 -> On Delay/1, Longitudinal Adjustments for Lane Change/3(lcFlag), Regular Vehicle Following/3(lcFlag)
  vlLeaderStates/1 -> Longitudinal Adjustments for Lane Change/2(leaderStates)
  leaderStates/1 -> Regular Vehicle Following/2(leaderStates)
  Bus Creator/1 -> Longitudinal Adjustments for Lane Change/1(currentStates), Regular Vehicle Following/1(currentStates), states/1
  Regular Vehicle Following/3(gap) -> gap/1
  Mux1/1 -> Terminator/1
  Vehicle Body 3DOF Single Track/7 -> Mux1/6
  Vehicle Body 3DOF Single Track/6 -> Mux1/5
  Vehicle Body 3DOF Single Track/5 -> Mux1/4
  Vehicle Body 3DOF Single Track/2 -> Mux1/1
  Vehicle Body 3DOF Single Track/3 -> Mux1/2
  Vehicle Body 3DOF Single Track/4 -> Mux1/3
  Vehicle Body 3DOF Single Track/1 -> Bus Selector/1
  Gain/1 -> Vehicle Body 3DOF Single Track/2, Vehicle Body 3DOF Single Track/3
  Bus Selector/1 -> Bus Creator/1  "<X>"
  Bus Selector/3 -> Bus Creator/3  "<Xdot>"

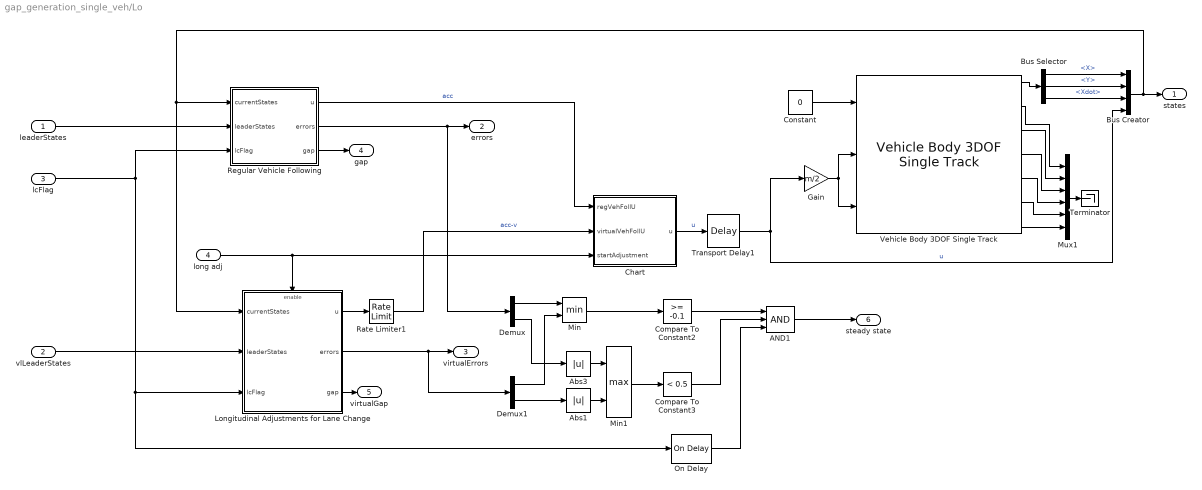
== system gap_generation_single_veh/Lo ==
  leaderStates : Inport
  vlLeaderStates : Inport  Port=2
  lcFlag : Inport  Port=3
  long adj : Inport  Port=4
  AND1 : Logic  Inputs=3  IconShape=distinctive  AllPortsSameDT=off  OutDataTypeStr=boolean
  Abs1 : Abs
  Abs3 : Abs
  Bus Creator : BusCreator  Inputs=4
  Bus Selector : BusSelector  OutputSignals=InertFrm.RearAxl.Disp.X,InertFrm.RearAxl.Disp.Y,InertFrm.RearAxl.Vel.Xdot
  Chart : Stateflow chart  BlockKeywords=__PRM__SERIALIZED__DATA__:Stateflow Chart,Stateflow Diagram  TreatAsAtomicUnit=on
  Compare To Constant2 : simulink/Logic and Bit Operations/Compare To Constant  relop=>=  const=-0.1  OutDataTypeStr=boolean
  Compare To Constant3 : simulink/Logic and Bit Operations/Compare To Constant  relop=<  const=0.5  OutDataTypeStr=boolean
  Constant : Constant  Value=0
  Demux : Demux  Outputs=2
  Demux1 : Demux  Outputs=2
  Gain : Gain  Gain=m/2
  Longitudinal Adjustments for Lane Change : Subsystem  TreatAsAtomicUnit=on
  Min : MinMax  Inputs=2
  Min1 : MinMax  Function=max  Inputs=2
  Mux1 : Mux  Inputs=6
  On Delay : powerlib_meascontrol/Logic/On Delay  DelayType=On delay  delay=1  ic=0  Ts=0
      settings: SourceProductName=Simscape Electrical
  Rate Limiter1 : RateLimiter  RisingSlewLimit=10  FallingSlewLimit=-10  SampleTimeMode=inherited
  Regular Vehicle Following : Subsystem
  Terminator : Terminator
  Transport Delay1 : TransportDelay  DelayTime=0.01
  Vehicle Body 3DOF Single Track : autolibshared/Vehicle Body 3DOF Single Track  trackMode=Single (bicycle)  inputMode=External longitudinal forces  frontSteerMode=on  rearSteerMode=off  windMode=off  muMode=off  extFMode=off  extMMode=off  extXo=off  extpsio=off  extxdoto=off  extro=off  extYo=off  extTamb=off  extydoto=off  aMode=2  NF=2  NR=2  m=m  a=lf  b=lr  h=0.35  X_o=x0  xdot_o=vx0  CalphaMode=off  sigmaMode=on  d=0  w=[1.4,1.4]  Cy_f=12e3  Cy_r=11e3  sigma_f=.1  sigma_r=.1  alpha_f_brk=[-.1 .1]  Cy_f_data=[-9e3 9e3]  alpha_r_brk=[-.1 .1]  Cy_r_data=[-9e3 9e3]  Y_o=y0  ydot_o=0  Izz=4000  psi_o=0  r_o=0  Af=2  Cd=.3  Cl=.1  Cpm=.1  beta_w=[0:0.01:0.3]  Cs=[0:0.03:0.9]  Cym=[0:0.01:0.3]  Pabs=101325  Tair=273  g=9.81  mu=1  xdot_tol=.01  Fznom=5000  Fxtire_sat=7e4  Fytire_sat=7e4  longOff=0  latOff=0  vertOff=0  wrapAng=off
      settings: SourceProductName=Powertrain Blockset  SourceProductBaseCode=PW
  states : Outport
  errors : Outport  Port=2
  virtualErrors : Outport  Port=3
  gap : Outport  Port=4
  virtualGap : Outport  Port=5
  steady state : Outport  Port=6
  wires:
  Constant/1 -> Vehicle Body 3DOF Single Track/1
  Bus Selector/2 -> Bus Creator/2  "<Y>"
  Abs1/1 -> Min1/2
  Abs3/1 -> Min1/1
  Longitudinal Adjustments for Lane Change/2(errors) -> Demux1/1, virtualErrors/1
  Min1/1 -> Compare To Constant3/1
  Compare To Constant3/1 -> AND1/2
  Compare To Constant2/1 -> AND1/1
  Demux1/2 -> Abs1/1
  Demux/2 -> Abs3/1
  Demux1/1 -> Min/2
  Demux/1 -> Min/1
  Min/1 -> Compare To Constant2/1
  Regular Vehicle Following/2(errors) -> Demux/1, errors/1
  Transport Delay1/1 -> Gain/1, Bus Creator/4  "u"
  Chart/1(u) -> Transport Delay1/1  "u"
  Rate Limiter1/1 -> Chart/2(virtualVehFollU)  "acc-v"
  Regular Vehicle Following/1(u) -> Chart/1(regVehFollU)  "acc"
  Longitudinal Adjustments for Lane Change/1(u) -> Rate Limiter1/1
  AND1/1 -> steady state/1
  On Delay/1 -> AND1/3
  long adj/1 -> Longitudinal Adjustments for Lane Change/Enable, Chart/3(startAdjustment)
  Longitudinal Adjustments for Lane Change/3(gap) -> virtualGap/1
  lcFlag/1 -> On Delay/1, Longitudinal Adjustments for Lane Change/3(lcFlag), Regular Vehicle Following/3(lcFlag)
  vlLeaderStates/1 -> Longitudinal Adjustments for Lane Change/2(leaderStates)
  leaderStates/1 -> Regular Vehicle Following/2(leaderStates)
  Bus Creator/1 -> Longitudinal Adjustments for Lane Change/1(currentStates), Regular Vehicle Following/1(currentStates), states/1
  Regular Vehicle Following/3(gap) -> gap/1
  Mux1/1 -> Terminator/1
  Vehicle Body 3DOF Single Track/7 -> Mux1/6
  Vehicle Body 3DOF Single Track/6 -> Mux1/5
  Vehicle Body 3DOF Single Track/5 -> Mux1/4
  Vehicle Body 3DOF Single Track/2 -> Mux1/1
  Vehicle Body 3DOF Single Track/3 -> Mux1/2
  Vehicle Body 3DOF Single Track/4 -> Mux1/3
  Vehicle Body 3DOF Single Track/1 -> Bus Selector/1
  Gain/1 -> Vehicle Body 3DOF Single Track/2, Vehicle Body 3DOF Single Track/3
  Bus Selector/1 -> Bus Creator/1  "<X>"
  Bus Selector/3 -> Bus Creator/3  "<Xdot>"

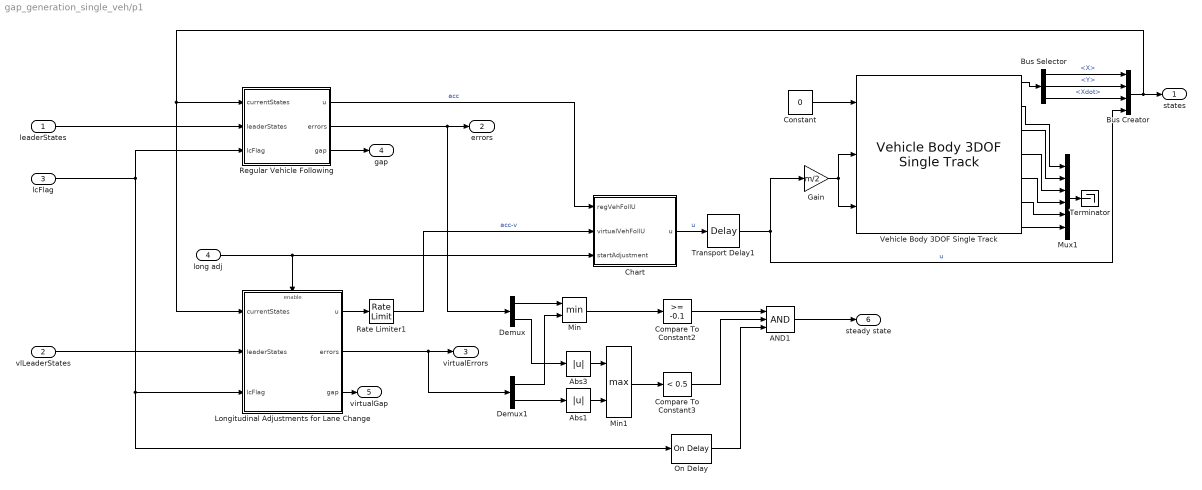
== system gap_generation_single_veh/p1 ==
  leaderStates : Inport
  vlLeaderStates : Inport  Port=2
  lcFlag : Inport  Port=3
  long adj : Inport  Port=4
  AND1 : Logic  Inputs=3  IconShape=distinctive  AllPortsSameDT=off  OutDataTypeStr=boolean
  Abs1 : Abs
  Abs3 : Abs
  Bus Creator : BusCreator  Inputs=4
  Bus Selector : BusSelector  OutputSignals=InertFrm.RearAxl.Disp.X,InertFrm.RearAxl.Disp.Y,InertFrm.RearAxl.Vel.Xdot
  Chart : Stateflow chart  BlockKeywords=__PRM__SERIALIZED__DATA__:Stateflow Chart,Stateflow Diagram  TreatAsAtomicUnit=on
  Compare To Constant2 : simulink/Logic and Bit Operations/Compare To Constant  relop=>=  const=-0.1  OutDataTypeStr=boolean
  Compare To Constant3 : simulink/Logic and Bit Operations/Compare To Constant  relop=<  const=0.5  OutDataTypeStr=boolean
  Constant : Constant  Value=0
  Demux : Demux  Outputs=2
  Demux1 : Demux  Outputs=2
  Gain : Gain  Gain=m/2
  Longitudinal Adjustments for Lane Change : Subsystem  TreatAsAtomicUnit=on
  Min : MinMax  Inputs=2
  Min1 : MinMax  Function=max  Inputs=2
  Mux1 : Mux  Inputs=6
  On Delay : powerlib_meascontrol/Logic/On Delay  DelayType=On delay  delay=1  ic=0  Ts=0
      settings: SourceProductName=Simscape Electrical
  Rate Limiter1 : RateLimiter  RisingSlewLimit=10  FallingSlewLimit=-10  SampleTimeMode=inherited
  Regular Vehicle Following : Subsystem
  Terminator : Terminator
  Transport Delay1 : TransportDelay  DelayTime=0.01
  Vehicle Body 3DOF Single Track : autolibshared/Vehicle Body 3DOF Single Track  trackMode=Single (bicycle)  inputMode=External longitudinal forces  frontSteerMode=on  rearSteerMode=off  windMode=off  muMode=off  extFMode=off  extMMode=off  extXo=off  extpsio=off  extxdoto=off  extro=off  extYo=off  extTamb=off  extydoto=off  aMode=2  NF=2  NR=2  m=m  a=lf  b=lr  h=0.35  X_o=x0  xdot_o=vx0  CalphaMode=off  sigmaMode=on  d=0  w=[1.4,1.4]  Cy_f=12e3  Cy_r=11e3  sigma_f=.1  sigma_r=.1  alpha_f_brk=[-.1 .1]  Cy_f_data=[-9e3 9e3]  alpha_r_brk=[-.1 .1]  Cy_r_data=[-9e3 9e3]  Y_o=y0  ydot_o=0  Izz=4000  psi_o=0  r_o=0  Af=2  Cd=.3  Cl=.1  Cpm=.1  beta_w=[0:0.01:0.3]  Cs=[0:0.03:0.9]  Cym=[0:0.01:0.3]  Pabs=101325  Tair=273  g=9.81  mu=1  xdot_tol=.01  Fznom=5000  Fxtire_sat=7e4  Fytire_sat=7e4  longOff=0  latOff=0  vertOff=0  wrapAng=off
      settings: SourceProductName=Powertrain Blockset  SourceProductBaseCode=PW
  states : Outport
  errors : Outport  Port=2
  virtualErrors : Outport  Port=3
  gap : Outport  Port=4
  virtualGap : Outport  Port=5
  steady state : Outport  Port=6
  wires:
  Constant/1 -> Vehicle Body 3DOF Single Track/1
  Bus Selector/2 -> Bus Creator/2  "<Y>"
  Abs1/1 -> Min1/2
  Abs3/1 -> Min1/1
  Longitudinal Adjustments for Lane Change/2(errors) -> Demux1/1, virtualErrors/1
  Min1/1 -> Compare To Constant3/1
  Compare To Constant3/1 -> AND1/2
  Compare To Constant2/1 -> AND1/1
  Demux1/2 -> Abs1/1
  Demux/2 -> Abs3/1
  Demux1/1 -> Min/2
  Demux/1 -> Min/1
  Min/1 -> Compare To Constant2/1
  Regular Vehicle Following/2(errors) -> Demux/1, errors/1
  Transport Delay1/1 -> Gain/1, Bus Creator/4  "u"
  Chart/1(u) -> Transport Delay1/1  "u"
  Rate Limiter1/1 -> Chart/2(virtualVehFollU)  "acc-v"
  Regular Vehicle Following/1(u) -> Chart/1(regVehFollU)  "acc"
  Longitudinal Adjustments for Lane Change/1(u) -> Rate Limiter1/1
  AND1/1 -> steady state/1
  On Delay/1 -> AND1/3
  long adj/1 -> Longitudinal Adjustments for Lane Change/Enable, Chart/3(startAdjustment)
  Longitudinal Adjustments for Lane Change/3(gap) -> virtualGap/1
  lcFlag/1 -> On Delay/1, Longitudinal Adjustments for Lane Change/3(lcFlag), Regular Vehicle Following/3(lcFlag)
  vlLeaderStates/1 -> Longitudinal Adjustments for Lane Change/2(leaderStates)
  leaderStates/1 -> Regular Vehicle Following/2(leaderStates)
  Bus Creator/1 -> Longitudinal Adjustments for Lane Change/1(currentStates), Regular Vehicle Following/1(currentStates), states/1
  Regular Vehicle Following/3(gap) -> gap/1
  Mux1/1 -> Terminator/1
  Vehicle Body 3DOF Single Track/7 -> Mux1/6
  Vehicle Body 3DOF Single Track/6 -> Mux1/5
  Vehicle Body 3DOF Single Track/5 -> Mux1/4
  Vehicle Body 3DOF Single Track/2 -> Mux1/1
  Vehicle Body 3DOF Single Track/3 -> Mux1/2
  Vehicle Body 3DOF Single Track/4 -> Mux1/3
  Vehicle Body 3DOF Single Track/1 -> Bus Selector/1
  Gain/1 -> Vehicle Body 3DOF Single Track/2, Vehicle Body 3DOF Single Track/3
  Bus Selector/1 -> Bus Creator/1  "<X>"
  Bus Selector/3 -> Bus Creator/3  "<Xdot>"

== system gap_generation_single_veh/Fd/Longitudinal Adjustments for Lane Change ==
  currentStates : Inport
  leaderStates : Inport  Port=2
  lcFlag : Inport  Port=3
  Enable : EnablePort
  Bus Selector : BusSelector  OutputSignals=X,Xdot,u
  Bus Selector1 : BusSelector  OutputSignals=X,Xdot
  Chart : Stateflow chart  BlockKeywords=__PRM__SERIALIZED__DATA__:Stateflow Chart,Stateflow Diagram  TreatAsAtomicUnit=on
  Gain3 : Gain  Gain=velFilterGain/10
  Headway error : Subsystem
  Input Saturation : Saturate  UpperLimit=maxComfAccel  LowerLimit=minComfAccel
  Integrator1 : Integrator  InitialCondition=vx0
  Mux : Mux  Inputs=2
  Rate Limiter : RateLimiter  RisingSlewLimit=maxComfJerk  FallingSlewLimit=minComfJerk  SampleTimeMode=inherited
  Saturation : Saturate  UpperLimit=maxAcceleration  LowerLimit=minAcceleration
  Scope3 : Scope  NumInputPorts=2
  Sum : Sum  Inputs=-+|
  Sum2 : Sum  Inputs=|+-
  Sum6 : Sum  Inputs=|+-
  Transport Delay : TransportDelay  DelayTime=0.01
  Transport Delay1 : TransportDelay  DelayTime=0.01
  Veh Following : Subsystem  TreatAsAtomicUnit=on
  Velocity Control : Subsystem  TreatAsAtomicUnit=on
  vMin : Constant  Value=vMin
  u : Outport  InitialOutput=0
  errors : Outport  Port=2  OutputWhenDisabled=reset  InitialOutput=[0, 0]
  gap : Outport  Port=3  OutputWhenDisabled=reset  InitialOutput=[0]
  wires:
  Bus Selector/3 -> Veh Following/3(realInput)  "<u>"
  lcFlag/1 -> Headway error/4(lcFlag)
  Bus Selector1/1 -> Headway error/3(xl)  "<X>"
  leaderStates/1 -> Bus Selector1/1
  Headway error/2("gap ") -> gap/1
  currentStates/1 -> Bus Selector/1
  Bus Selector/1 -> Headway error/1(xf)  "<X>"
  Bus Selector/2 -> Headway error/2(vf), Sum/1, Sum6/2  "<Xdot>"
  Mux/1 -> errors/1
  Integrator1/1 -> Sum/2, Sum2/2
  Gain3/1 -> Saturation/1
  vMin/1 -> Sum6/1
  Sum/1 -> Mux/2, Veh Following/2(ev)  "ev"
  Chart/2(u) -> Transport Delay/1  "u"
  Bus Selector1/2 -> Sum2/1  "<Xdot>"
  Sum6/1 -> Chart/1(velDiff), Velocity Control/2(ev)
  Sum2/1 -> Gain3/1
  Headway error/1(eh) -> Mux/1, Veh Following/1(eh)  "eh"
  Rate Limiter/1 -> u/1, Scope3/2  "sat(u)"
  Input Saturation/1 -> Rate Limiter/1
  Saturation/1 -> Integrator1/1
  Veh Following/1(u) -> Chart/3(uVehFoll)  "uVehFoll"
  Velocity Control/1(Out1) -> Chart/2(uVelControl)  "uVelControl"
  Transport Delay/1 -> Input Saturation/1, Scope3/1
  Chart/1(state) -> Transport Delay1/1
  Transport Delay1/1 -> Velocity Control/1(intReset)

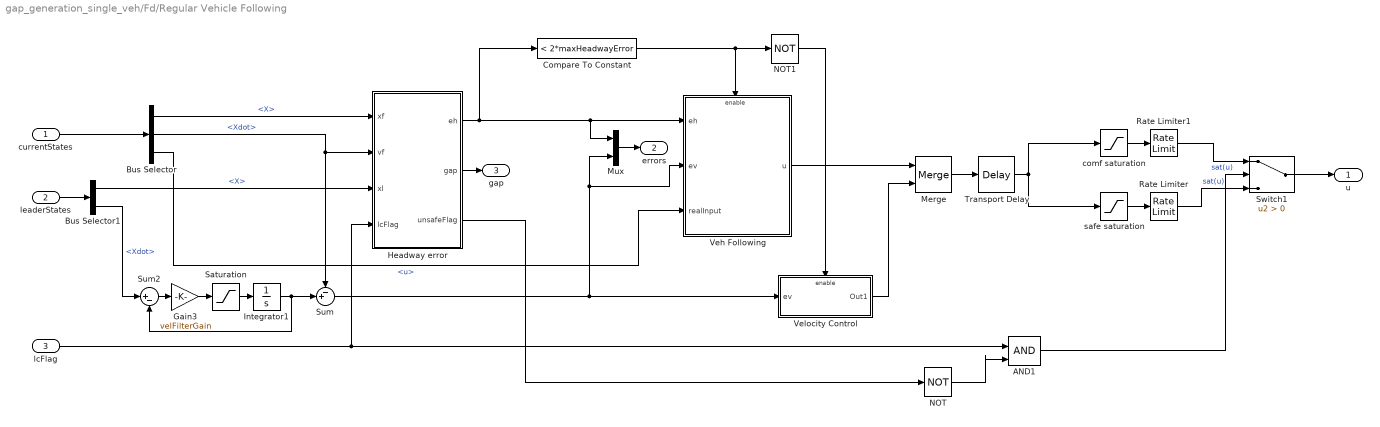
== system gap_generation_single_veh/Fd/Regular Vehicle Following ==
  currentStates : Inport
  leaderStates : Inport  Port=2
  lcFlag : Inport  Port=3
  AND1 : Logic  IconShape=distinctive  AllPortsSameDT=off  OutDataTypeStr=boolean
  Bus Selector : BusSelector  OutputSignals=X,Xdot,u
  Bus Selector1 : BusSelector  OutputSignals=X,Xdot
  Compare To Constant : simulink/Logic and Bit Operations/Compare To Constant  relop=<  const=2*maxHeadwayError  OutDataTypeStr=boolean
  Gain3 : Gain  Gain=velFilterGain
  Headway error : Subsystem
  Integrator1 : Integrator  InitialCondition=vx0
  Merge : Merge
  Mux : Mux  Inputs=2
  NOT : Logic  Operator=NOT  IconShape=distinctive  AllPortsSameDT=off  OutDataTypeStr=boolean
  NOT1 : Logic  Operator=NOT  IconShape=distinctive  AllPortsSameDT=off  OutDataTypeStr=boolean
  Rate Limiter : RateLimiter  RisingSlewLimit=maxJerk  FallingSlewLimit=minJerk  SampleTimeMode=inherited
  Rate Limiter1 : RateLimiter  RisingSlewLimit=maxComfJerk  FallingSlewLimit=minComfJerk  SampleTimeMode=inherited
  Saturation : Saturate  UpperLimit=maxAcceleration  LowerLimit=minAcceleration
  Sum : Sum  Inputs=-+|
  Sum2 : Sum  Inputs=|+-
  Switch1 : Switch  Criteria=u2 > Threshold
  Transport Delay : TransportDelay  DelayTime=0.01
  Veh Following : Subsystem  TreatAsAtomicUnit=on
  Velocity Control : Subsystem  TreatAsAtomicUnit=on
  comf saturation : Saturate  UpperLimit=maxComfAccel  LowerLimit=minComfAccel
  safe saturation : Saturate  UpperLimit=maxAcceleration  LowerLimit=minAcceleration
  u : Outport
  errors : Outport  Port=2
  gap : Outport  Port=3
  wires:
  Bus Selector/2 -> Sum/1, Headway error/2(vf)  "<Xdot>"
  Gain3/1 -> Saturation/1
  Saturation/1 -> Integrator1/1
  Integrator1/1 -> Sum2/2, Sum/2
  Bus Selector1/2 -> Sum2/1  "<Xdot>"
  Sum2/1 -> Gain3/1
  Sum/1 -> Mux/2, Veh Following/2(ev), Velocity Control/1(ev)
  currentStates/1 -> Bus Selector/1
  Bus Selector/1 -> Headway error/1(xf)  "<X>"
  leaderStates/1 -> Bus Selector1/1
  comf saturation/1 -> Rate Limiter1/1
  AND1/1 -> Switch1/2
  safe saturation/1 -> Rate Limiter/1
  Rate Limiter/1 -> Switch1/3  "sat(u)"
  Switch1/1 -> u/1
  Rate Limiter1/1 -> Switch1/1  "sat(u)"
  Veh Following/1(u) -> Merge/1
  Compare To Constant/1 -> NOT1/1, Veh Following/Enable
  Velocity Control/1(Out1) -> Merge/2
  Merge/1 -> Transport Delay/1
  Transport Delay/1 -> safe saturation/1, comf saturation/1
  Mux/1 -> errors/1
  Headway error/1(eh) -> Mux/1, Veh Following/1(eh), Compare To Constant/1
  Headway error/2("gap ") -> gap/1
  Headway error/3(unsafeFlag) -> NOT/1
  Bus Selector1/1 -> Headway error/3(xl)  "<X>"
  Bus Selector/3 -> Veh Following/3(realInput)  "<u>"
  NOT/1 -> AND1/2
  lcFlag/1 -> AND1/1, Headway error/4(lcFlag)
  NOT1/1 -> Velocity Control/Enable
